simulink model "problema1b"  (R2019a)
settings: Solver=FixedStepAuto  StartTime=0.0  StopTime=10.0  FixedStep=1  RelTol=1e-3
libraries: simulink x4
settings Model: Creator=prestamour  LastModifiedBy=prestamour

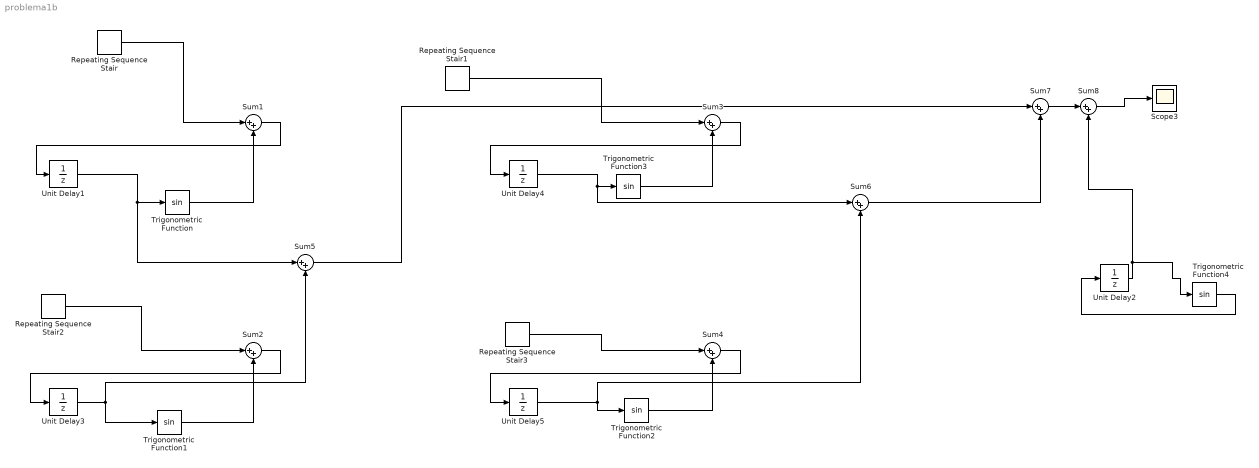
== system problema1b ==
  Repeating Sequence Stair : simulink/Sources/Repeating Sequence Stair  OutValues=[0 1 0 0 0 0 0 0 0 0 0 0].'  tsamp=-1  OutMin=[]  OutMax=[]  OutDataTypeStr=double  OutputDataTypeScalingMode=double  OutDataType=fixdt(0,8)  ConRadixGroup=Best Precision: Vector-wise  OutScaling=2^-12
  Repeating Sequence Stair1 : simulink/Sources/Repeating Sequence Stair  OutValues=[0 0 1 0 0 0 0 0 0 0 0 0].'  tsamp=-1  OutMin=[]  OutMax=[]  OutDataTypeStr=double  OutputDataTypeScalingMode=double  OutDataType=fixdt(0,8)  ConRadixGroup=Best Precision: Vector-wise  OutScaling=2^-12
  Repeating Sequence Stair2 : simulink/Sources/Repeating Sequence Stair  OutValues=[0 0 0 1 0 0 0 0 0 0 0 0].'  tsamp=-1  OutMin=[]  OutMax=[]  OutDataTypeStr=double  OutputDataTypeScalingMode=double  OutDataType=fixdt(0,8)  ConRadixGroup=Best Precision: Vector-wise  OutScaling=2^-12
  Repeating Sequence Stair3 : simulink/Sources/Repeating Sequence Stair  OutValues=[0 0 0 0 1 0 0 0 0 0 0 0].'  tsamp=-1  OutMin=[]  OutMax=[]  OutDataTypeStr=double  OutputDataTypeScalingMode=double  OutDataType=fixdt(0,8)  ConRadixGroup=Best Precision: Vector-wise  OutScaling=2^-12
  Scope3 : Scope
  Sum{1..8} (8 alike) : Sum  Inputs=|++
  Trigonometric Function{,1..4} (5 alike) : Trigonometry
  Unit Delay{1,3..5} (4 alike) : UnitDelay  SampleTime=-1  HasFrameUpgradeWarning=on
  Unit Delay2 : UnitDelay  InitialCondition=1  SampleTime=-1  HasFrameUpgradeWarning=on
  wires:
  Unit Delay3/1 -> Trigonometric Function1/1, Sum5/2
  Unit Delay5/1 -> Trigonometric Function2/1, Sum6/2
  Sum5/1 -> Sum7/1
  Repeating Sequence Stair2/1 -> Sum2/1
  Sum4/1 -> Unit Delay5/1
  Sum2/1 -> Unit Delay3/1
  Sum3/1 -> Unit Delay4/1
  Sum6/1 -> Sum7/2
  Repeating Sequence Stair1/1 -> Sum3/1
  Unit Delay4/1 -> Trigonometric Function3/1, Sum6/1
  Unit Delay1/1 -> Trigonometric Function/1, Sum5/1
  Repeating Sequence Stair3/1 -> Sum4/1
  Repeating Sequence Stair/1 -> Sum1/1
  Trigonometric Function/1 -> Sum1/2
  Trigonometric Function1/1 -> Sum2/2
  Trigonometric Function3/1 -> Sum3/2
  Trigonometric Function2/1 -> Sum4/2
  Unit Delay2/1 -> Trigonometric Function4/1, Sum8/2
  Trigonometric Function4/1 -> Unit Delay2/1
  Sum7/1 -> Sum8/1
  Sum8/1 -> Scope3/1
  Sum1/1 -> Unit Delay1/1
